simulink library "Pump_Const"  (R2018b)
settings: Solver=ode45  StartTime=0.0  StopTime=10.0  RelTol=1e-3  EnableMultiTasking=on
undefined symbols (not defined in the file): Water
libraries: carnot x3
settings Model: Creator=Hafner  LastModifiedBy=P41573
settings DataIOCC: LimitDataPoints=on  SaveFormat=Array  SignalLoggingSaveFormat=ModelDataLogs
settings OptimizationCC: ExpressionDepthLimit=2147483647  LifeSpan=inf
settings DebuggingCC: UnderspecifiedInitializationDetection=Classic  MergeDetectMultiDrivingBlocksExec=none  SolverPrmCheckMsg=warning  FcnCallInpInsideContextMsg=warning  StateNameClashWarn=warning  SFUnexpectedBacktrackingDiag=warning  SFNoUnconditionalDefaultTransitionDiag=warning  SFExecutionAtInitializationDiag=none
settings HardwareCC: ProdBitPerPointer=32  ProdBitPerSizeT=32  ProdBitPerPtrDiffT=32  ProdLargestAtomicFloat=None  ProdIntDivRoundTo=Undefined  ProdEndianess=Unspecified  ProdWordSize=32  ProdHWDeviceType=32-bit Generic
settings ModelReferenceCC: PropagateSignalLabelsOutOfModel=off
settings SFSimCC: SimUseLocalCustomCode=off
settings RTWCC: RTWUseLocalCustomCode=off
settings CodeAppCC: StateflowObjectComments=on
settings GRTTargetCC: TargetLangStandard=C89/C90 (ANSI)  GeneratePreprocessorConditionals=Disable all  CombineOutputUpdateFcns=off  GRTInterface=on
settings ConfigComp: CovMetricSettings=dw  CovHtmlReporting=on  CovSaveCumulativeToWorkspaceVar=on  CovSaveSingleToWorkspaceVar=on  CovExternalEMLEnable=off

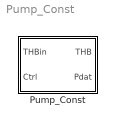
== system Pump_Const ==
  Pump_Const : Subsystem  mask(Pump constant){mdotmax=1200/3600, dia=0.02, p0=3e5, fluid_id=Water, mix=0, mix2=0, mix3=0, UA=3, mcp=4182, Tini=20, e0=10, e1=10, e2=-1}
      mask prompts: mdotmax "mdotmax : massflow rate in kg/s"; dia "diameter at in- and outlet [m]"; p0 "system pressure [Pa]"; fluid_id "fluid"; mix "percentage of fluid mix [0..1]"; mix2 "fluid mixture 2 [0..1]"; mix3 "fluid mixture 3 [0..1]"; UA "Thermal loss coefficient to ambient in W/K"; mcp "mcp: thermal capacity of the node in J/K"; Tini "Initial and ambient temperature in °C"; e0 "e0: constant coefficient in W"; e1 "e1: linear coefficient in W*s/kg"; e2 "e2: quadratic coefficient in W*(s/kg)²"
      mask help:
      | Set constant massflow rate according to the parameter mdotmax and the control signal:
      | mdot = mdotmax * Ctrl
      | Use the option "thermal node" if you want the pump to have thermal capacity and losses to ambient (or if you want to break an algebraic loop in the temperature signal).
      | Electric power is calculated Pel = e0 + e1*mdot + e2*mdot^2
      mask Help: web(fullfile(path_carnot('help'),'Pump_Const.html'),'-helpbrowser')
      mask TypeOptions mdotmax: Pump_basic/mdotmax
      mask TypeOptions dia: Pump_basic/dia
      mask TypeOptions p0: Pump_basic/p0
      mask TypeOptions fluid_id: Pump_basic/fluid_id
      mask TypeOptions mix: Pump_basic/mix
      mask TypeOptions mix2: Pump_basic/mix2
      mask TypeOptions mix3: Pump_basic/mix3
      mask TypeOptions UA: ThermalNodeTHB/UA
      mask TypeOptions mcp: ThermalNodeTHB/mcp
      mask TypeOptions Tini: ThermalNodeTHB/Tini
      mask TypeOptions e0: ElectricConsumptionPump/e0
      mask TypeOptions e1: ElectricConsumptionPump/e1
      mask TypeOptions e2: ElectricConsumptionPump/e2
      mask DialogControl ParameterTabVar0 Prompt: Hydraulic
      mask DialogControl ParameterTabVar012 Prompt: Thermal
      mask DialogControl ParameterTabVar01 Prompt: Electric
      mask Display:
      | plot(0,0,100,100,...
      |     [40,70,40,30,30,40,60,70,70,60,40],[70,50,30,40,60,70,70,60,40,30,30])

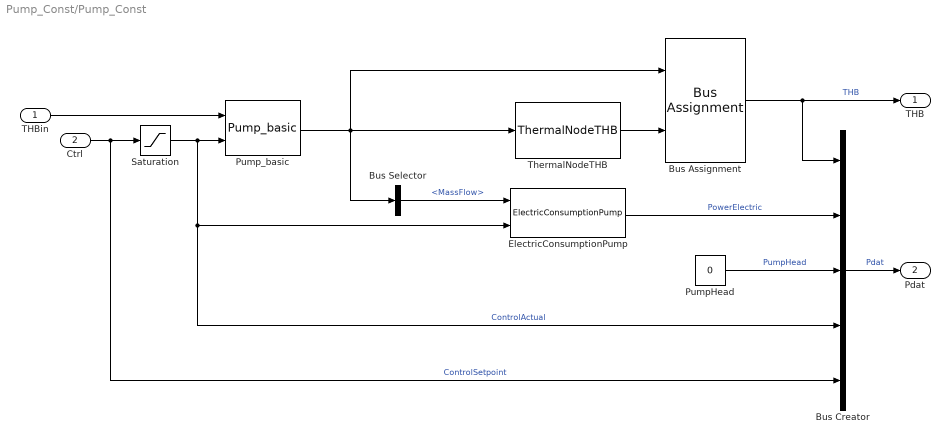
== system Pump_Const/Pump_Const ==
  THBin : Inport
  Ctrl : Inport  Port=2
  Bus Assignment : BusAssignment  AssignedSignals=Temperature
  Bus Creator : BusCreator  Inputs=5
  Bus Selector : BusSelector  OutputSignals=MassFlow
  ElectricConsumptionPump : carnot/Basic/Hydraulics/ElectricConsumptionPump  e0=e0  e1=e1  e2=e2
      settings: SourceProductName=Carnot
  PumpHead : Constant  Value=0
  Pump_basic : carnot/Hydraulics/Pump_basic  mdotmax=mdotmax  fluid_id=Water  mix=mix  mix2=mix2  mix3=mix3  p0=p0  dia=dia  ID=No Pressure Drop  hgt=0
      settings: SourceProductName=Carnot
  Saturation : Saturate  UpperLimit=1  LowerLimit=0
  ThermalNodeTHB : carnot/Basic/Thermal_Models/ThermalNodeTHB  UA=UA  mcp=mcp  Tini=Tini
      settings: SourceProductName=Carnot
  THB : Outport
  Pdat : Outport  Port=2
  wires:
  Bus Selector/1 -> ElectricConsumptionPump/1  "<MassFlow>"
  Ctrl/1 -> Saturation/1, Bus Creator/5  "ControlSetpoint"
  THBin/1 -> Pump_basic/1
  Pump_basic/1 -> Bus Assignment/1, Bus Selector/1, ThermalNodeTHB/1
  PumpHead/1 -> Bus Creator/3  "PumpHead"
  Bus Assignment/1 -> Bus Creator/1, THB/1  "THB"
  Bus Creator/1 -> Pdat/1  "Pdat"
  ElectricConsumptionPump/1 -> Bus Creator/2  "PowerElectric"
  Saturation/1 -> Bus Creator/4, ElectricConsumptionPump/2, Pump_basic/2  "ControlActual"
  ThermalNodeTHB/1 -> Bus Assignment/2
